simulink model "DS_distrIntp_1_10_simulated axes"  (R2019a)
settings: Solver=FixedStepDiscrete  StartTime=0.0  StopTime=inf  FixedStep=Ts  RelTol=1e-3
InitFcn:
  | %% Verwende vordefinierte Setpoints (Kreis mit Z-Komponente)
  | 
  | % Config
  | numCircles = 3;
  | scale=6;
  | %Versuch symmetrische Setpunkte zu setzen
  | pointsPerCircle =scale*(4+3*numCircles)+2;
  | 
  | r = 50;
  | m_x = r;
  | m_y = r;
  | 
  | % //
  | s = linspace(0,2*pi,pointsPerCircle);
  | 
  | setPoints_x = [];
  | setPoints_y = [];
  | 
  | for ii=1:numCircles
  | 
  | setPoints_x = [setPoints_x (-cos(s(1:floor(pointsPerCircle / 2))).*r + m_x + 2*r*(ii-1))]; %#ok<AGROW>
  | setPoints_y = [setPoints_y (sin(s).*r+m_y)]; %#ok<AGROW>pointsPerCircle / 2
  | 
  | end
  | 
  | setPoints_x = [setPoints_x flip(setPoints_x(1:end))];
  | 
  | % Loeschen doppelter y-Werte (Kreisuebergang)
  | setPoints_x(pointsPerCircle .* [1:numCircles]) = [];
  | setPoints_y(pointsPerCircle .* [1:numCircles]) = [];
  | 
  | % setPoints_x= [linspace(0,setPoints_x(19),19) setPoints_x(20:end)];
  | % setPoints_y= [linspace(0,setPoints_y(19),19) setPoints_y(20:end)];
  | 
  | % Array Elemente verschieben
  | % setPoints_x = circshift(setPoints_x,-pointsPerCircle/4,2);
  | % setPoints_y = circshift(setPoints_y,-pointsPerCircle/4,2);
  | 
  | z = zeros(1,size(setPoints_x,2));
  | z_x = -5:5;
  | z_y = -z_x.^2 + 25;
  | z_idx = 90;
  | z_idx2 = 210;
  | z(z_idx:z_idx+length(z_x)-1) = z_y;
  | z(z_idx2:z_idx2+length(z_x)-1) = z_y;
  | % z = [z_y z];
  | setPoints_z = z;
  | 
  | % setPoints_x = [zeros(1,length(z_y)) setPoints_x];
  | % setPoints_y = [setPoints_y(1,1)*ones(1,length(z_y)) setPoints_y];
  | 
  | % Umrechnung der Einheiten für Demonstrator
  | % setPoints_x = setPoints_x ./ 1000;
  | % setPoints_y = setPoints_y ./ 1000;
  | % setPoints_z = setPoints_z ./ 1000;
  | 
  | 
  | %{
  | plot(setPoints_x,setPoints_y);
  | fig = figure;
  | ... (+13 lines)
StartFcn:
  | close all;
model workspace (MAT data in the model file):
  MCOS : class17 (value not decoded)
  MCOS : class17 (value not decoded)
  MCOS : class17 (value not decoded)
  MCOS : class17 (value not decoded)
  MCOS : class17 (value not decoded)
  MCOS : class17 (value not decoded)
  MCOS : class17 (value not decoded)
  MCOS : class17 (value not decoded)
  MCOS : class17 (value not decoded)
  MCOS : class17 (value not decoded)
  MCOS : class17 (value not decoded)
  MCOS : class17 (value not decoded)
  MCOS : class17 (value not decoded)
  MCOS : class17 (value not decoded)
undefined symbols (not defined in the file or in its folder): DiscIntNeverNeededParam, VelOverride
libraries: simulink x19, vrlib x5, sldrtlib x2
(part 4 of 4)

== stateflow chart DS_distrIntp_1_10_simulated axes/PosTracer_v2 ==
  state Create_Plot
    entry:
    startPos = DS_createTracePlot(numAxes);
  state Fetch_Positions
    entry:
    for ii=1:size(GET_istPos,1)
    switch ii
    case 1
    pos_x = GET_istPos(ii);
    case 2
    pos_y = GET_istPos(ii);
    case 3
    pos_z = GET_istPos(ii);
    end
    end
  state Update_Plot
    entry:
    if numAxes == 2
    DS_updateTracePlot(numAxes,pos_x+startPos(1,1),pos_y+startPos(1,2),0,false);
    elseif numAxes == 3
    DS_updateTracePlot(numAxes,pos_x+startPos(1,1),pos_y+startPos(1,2),...
    pos_z+startPos(1,3),true);
    end
  (default) -> Create_Plot
  Create_Plot -> Fetch_Positions
  Fetch_Positions -> Update_Plot
  Update_Plot -> Fetch_Positions : after(35,tick)
  data: numAx function_input; sPos function_output; numAx function_input; pos1 function_input; pos2 function_input; pos3 function_input; drawLine function_input; numAxes parameter; pos_x local =0; pos_y local =0; GET_istPos data_store_memory; pos_z local =0; startPos local size=[1 numAxes] =zeros(1,numAxes); ii local
  function sPos  = DS_createTracePlot(numAx):
    | function sPos  = DS_createTracePlot(numAx)
    | 
    | coder.extrinsic('evalin');
    | coder.extrinsic('setappdata');
    | 
    | setP = evalin('base','setP_mat');
    | 
    | sPos = zeros(1,numAx);
    | 
    | if(numAx == 3)
    |     fig = figure;
    |     ax = axes;
    |         
    |     [~,dim2,~] = size(setP);
    |     plot3(ax,setP(1,1:dim2),setP(2,1:dim2),setP(3,1:dim2));
    |     
    |     set(fig,'Tag','TraceFig');
    |     set(ax,'Tag','TraceAxes');
    |     set(ax,'NextPlot','add');
    |     set(ax,'YDir','reverse');
    |     set(ax,'ZDir','reverse');
    |     
    |     sPos(1,1) = setP(1,1);
    |     sPos(1,2) = setP(2,1);
    |     sPos(1,3) = setP(3,1);
    |     
    |     traceLine = plot3(ax,[setP(1,1) setP(1,1)],[setP(2,1) setP(2,1)],[setP(3,1) setP(3,1)],'Color',[0 0 1],'LineWidth',1);
    |     setappdata(ax,'traceLine',traceLine);
    |     
    | elseif(numAx == 2)
    |     
    |     fig = figure;
    |     ax = axes;
    |         
    |     [~,dim2] = size(setP);
    |     plot(ax,setP(1,1:dim2),setP(2,1:dim2));
    |     
    |     set(fig,'Tag','TraceFig');
    |     set(ax,'Tag','TraceAxes');
    |     set(ax,'NextPlot','add');
    |     
    |     sPos(1,1) = setP(1,1);
    |     sPos(1,2) = setP(2,1);
    |     
    |     traceLine = plot(ax,[setP(1,1) setP(1,1)],[setP(2,1) setP(2,1)],'Color',[0 0 1],'LineWidth',1);
    |     setappdata(ax,'traceLine',traceLine);
    |     
    | end
    | 
    | 
    | end
  function DS_updateTracePlot(numAx,pos1,pos2,pos3,drawLine):
    | function DS_updateTracePlot(numAx,pos1,pos2,pos3,drawLine)
    | 
    | coder.extrinsic('delete');
    | coder.extrinsic('scatter');
    | coder.extrinsic('scatter3');
    | coder.extrinsic('getappdata');
    | coder.extrinsic('setappdata');
    | 
    | ax = findobj('Tag','TraceAxes');
    | 
    | punkt = getappdata(ax,'tracePunkt');
    | 
    | if ~isempty(punkt)
    |     delete(punkt);
    | end
    | 
    | 
    | if(numAx == 3)
    |     
    |     punkt = scatter3(ax,pos1,pos2,pos3,'MarkerEdgeColor','r','LineWidth',2);
    |     setappdata(ax,'tracePunkt',punkt);
    |     
    |     if drawLine
    |         
    |         traceLine = getappdata(ax,'traceLine');
    |         XData = get(traceLine,'XData');
    |         YData = get(traceLine,'YData');
    |         ZData = get(traceLine,'ZData');
    |         
    |         set(traceLine,'XData',[XData pos1]);
    |         set(traceLine,'YData',[YData pos2]);
    |         set(traceLine,'ZData',[ZData pos3]);
    |         
    |     end
    |     
    | elseif(numAx == 2)
    |     
    |     punkt = scatter(ax,pos1,pos2,'MarkerEdgeColor','r','LineWidth',2);
    |     setappdata(ax,'tracePunkt',punkt);
    |     
    |     if drawLine
    |         
    |         traceLine = getappdata(ax,'traceLine');
    |         XData = get(traceLine,'XData');
    |         YData = get(traceLine,'YData');
    |         
    |         set(traceLine,'XData',[XData pos1]);
    |         set(traceLine,'YData',[YData pos2]);
    |         
    |     end
    |     
    | end
    | 
    | 
    | end

== stateflow chart DS_distrIntp_1_10_simulated axes/PosTracer_v1 ==
  state Create_Plot
    entry:
    startPos = DS_createTracePlot(numAxes);
  state Idle
    during:
    if numAxes == 2
    pos_x = GET_istPos(1);
    pos_y = GET_istPos(2);
    if pos_x ~= old_pos_x
    send(updated_pos);
    end
    if pos_y ~= old_pos_y
    send(updated_pos);
    end
    old_pos_x = pos_x;
    old_pos_y = pos_y;
    elseif numAxes == 3
    pos_x = GET_istPos(1);
    pos_y = GET_istPos(2);
    pos_z = GET_istPos(3);
    if pos_x ~= old_pos_x
    send(updated_pos);
    end
    if pos_y ~= old_pos_y
    send(updated_pos);
    end
    if pos_z ~= old_pos_z
    send(updated_pos);
    end
    old_pos_x = pos_x;
    old_pos_y = pos_y;
    old_pos_z = pos_z;
    end
  state Update_Plot
    entry:
    if numAxes == 2
    DS_updateTracePlot(numAxes,pos_x+startPos(1,1),pos_y+startPos(1,2),0);
    elseif numAxes == 3
    DS_updateTracePlot(numAxes,pos_x+startPos(1,1),pos_y+startPos(1,2),...
    pos_z+startPos(1,3));
    end
  (default) -> Create_Plot
  Create_Plot -> Idle
  Idle -> Update_Plot : updated_pos ...
      | {old_pos_x = pos_x; ...
      | old_pos_y = pos_y; ...
      | old_pos_z = pos_z}
  Update_Plot -> Idle : after(50,tick)
  data: numAx function_input; sPos function_output; numAx function_input; pos1 function_input; pos2 function_input; pos3 function_input; numAxes parameter; pos_x local =0; pos_y local =0; GET_istPos data_store_memory; pos_z local =0; old_pos_x local =0; old_pos_y local =0; old_pos_z local =0; startPos local size=[1 numAxes] =zeros(1,numAxes)
  events: updated_pos local FUNCTION_CALL_EVENT
  function sPos  = DS_createTracePlot(numAx):
    | function sPos  = DS_createTracePlot(numAx)
    | 
    | coder.extrinsic('evalin');
    | 
    | setP = evalin('base','setP_mat');
    | 
    | sPos = zeros(1,numAx);
    | 
    | if(numAx == 3)
    |     fig = figure;
    |     ax = axes;
    |         
    |     [~,dim2,~] = size(setP);
    |     plot3(ax,setP(1,1:dim2),setP(2,1:dim2),setP(3,1:dim2));
    |     
    |     set(fig,'Tag','TraceFig');
    |     set(ax,'Tag','TraceAxes');
    |     set(ax,'NextPlot','add');
    |     
    |     sPos(1,1) = setP(1,1);
    |     sPos(1,2) = setP(2,1);
    |     sPos(1,3) = setP(3,1);
    |     
    |     
    | end
    | 
    | 
    | end
  function DS_updateTracePlot(numAx,pos1,pos2,pos3):
    | function DS_updateTracePlot(numAx,pos1,pos2,pos3)
    | 
    | coder.extrinsic('delete');
    | coder.extrinsic('scatter3');
    | coder.extrinsic('getappdata');
    | coder.extrinsic('setappdata');
    | 
    | ax = findobj('Tag','TraceAxes');
    | 
    | punkt = getappdata(ax,'tracePunkt');
    | 
    | if ~isempty(punkt)
    |     delete(punkt);
    | end
    | 
    | 
    | if(numAx == 3)
    | 
    |    punkt = scatter3(ax,pos1,pos2,pos3,'MarkerEdgeColor','r','LineWidth',2);
    |    setappdata(ax,'tracePunkt',punkt);
    |    
    | end
    | 
    | 
    | end

== stateflow chart DS_distrIntp_1_10_simulated axes/Joystick Ctrl/Fetch_Global_Data/Chart ==
  state LeseVelOverride
    during:
    vel_x = abs(GET_velocity(1) / (10 * 0.8));
    vel_y = abs(GET_velocity(2) / (5 * 0.8));
    vel_z = abs(GET_velocity(3) / (2 * 0.8));
    velOR_x = VelOverride(1);
    velOR_y = VelOverride(2);
    velOR_z = VelOverride(3);
  (default) -> LeseVelOverride
  data: velOR_x output; velOR_y output; velOR_z output; VelOverride data_store_memory; GET_velocity data_store_memory; vel_x output; vel_y output; vel_z output
